simulink model "LKA_Driver_Switch"  (R2016a)
settings: Solver=VariableStepAuto  StartTime=0.0  StopTime=10.0  RelTol=1e-3
settings Model: Creator=91602  LastModifiedBy=91602

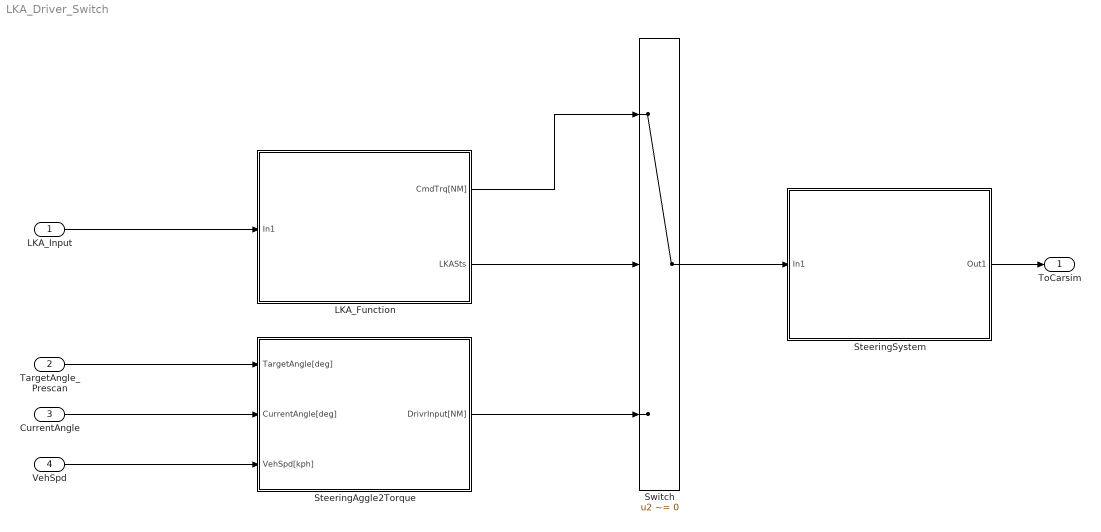
== system LKA_Driver_Switch ==
  LKA_Input : Inport
  TargetAngle_Prescan : Inport  Port=2
  CurrentAngle : Inport  Port=3
  VehSpd : Inport  Port=4
  LKA_Function : Subsystem
  SteeringAggle2Torque : Subsystem
  SteeringSystem : Subsystem
  Switch : Switch  Criteria=u2 ~= 0
  ToCarsim : Outport
  wires:
  TargetAngle_Prescan/1 -> SteeringAggle2Torque/1(TargetAngle[deg])
  CurrentAngle/1 -> SteeringAggle2Torque/2(CurrentAngle[deg])
  VehSpd/1 -> SteeringAggle2Torque/3(VehSpd[kph])
  LKA_Input/1 -> LKA_Function/1(In1)
  Switch/1 -> SteeringSystem/1(In1)
  SteeringSystem/1(Out1) -> ToCarsim/1
  LKA_Function/2(LKASts) -> Switch/2
  LKA_Function/1(CmdTrq[NM]) -> Switch/1
  SteeringAggle2Torque/1(DrivrInput[NM]) -> Switch/3

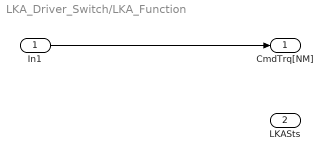
== system LKA_Driver_Switch/LKA_Function ==
  In1 : Inport
  CmdTrq[NM] : Outport
  LKASts : Outport  Port=2
  wires:
  In1/1 -> CmdTrq[NM]/1

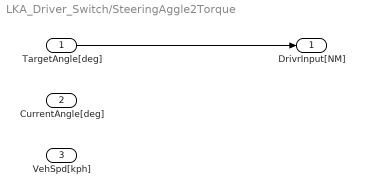
== system LKA_Driver_Switch/SteeringAggle2Torque ==
  TargetAngle[deg] : Inport
  CurrentAngle[deg] : Inport  Port=2
  VehSpd[kph] : Inport  Port=3
  DrivrInput[NM] : Outport
  wires:
  TargetAngle[deg]/1 -> DrivrInput[NM]/1

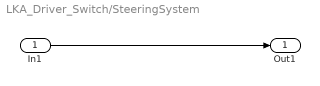
== system LKA_Driver_Switch/SteeringSystem ==
  In1 : Inport
  Out1 : Outport
  wires:
  In1/1 -> Out1/1
